simulink model "HeadwayControl_CleanedUpVFinal"  (R2018a)
settings: Solver=ode45  StartTime=0.0  StopTime=tsim  MaxStep=.1  RelTol=1e-3
values from neighbouring files (symbols this model uses):
  EndVel = (Time2-Time1)*Slope+StartVel    (= 31.525)    [ImpulseResponseStringStabilityV2.m]
  h = 2    [ImpulseResponseStringStabilityV2.m]
  InputNum = 3    [ImpulseResponseStringStabilityV2.m]
  InputTime = 1    [ImpulseResponseStringStabilityV2.m]
  lambda = 0.001    [ImpulseResponseStringStabilityV2.m]
  Slope = 0.5*g    (= 4.905)    [ImpulseResponseStringStabilityV2.m]
  StartVel = 7    [ImpulseResponseStringStabilityV2.m]
  tau = .5    (= 0.5)    [ImpulseResponseStringStabilityV2.m]
  Time1 = 2    [ImpulseResponseStringStabilityV2.m]
  Time2 = Time1 + DTime    (= 7)    [ImpulseResponseStringStabilityV2.m]
undefined symbols (not defined in the file or in its folder): heaviside
libraries: simulink x2
settings Model: Creator=domin  LastModifiedBy=domin

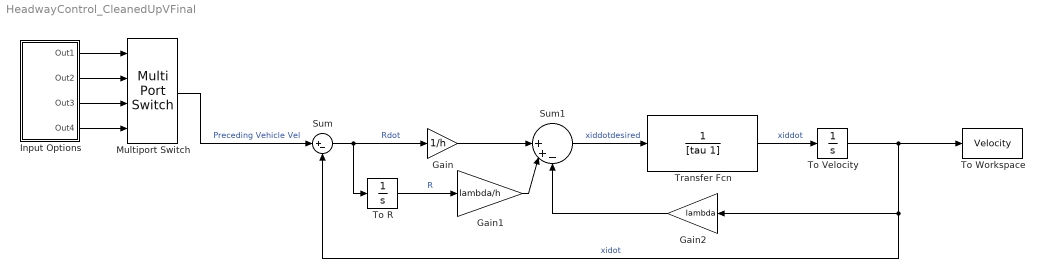
== system HeadwayControl_CleanedUpVFinal ==
  Gain : Gain  Gain=1/h
  Gain1 : Gain  Gain=lambda/h
  Gain2 : Gain  Gain=lambda
  Input Options : Subsystem
  Multiport Switch : MultiPortSwitch
  Sum : Sum  Inputs=|+-
  Sum1 : Sum  Inputs=||++-
  To R : Integrator  InitialCondition=h*StartVel
  To Velocity : Integrator  InitialCondition=StartVel
  To Workspace : ToWorkspace  VariableName=Velocity  SampleTime=-1
  Transfer Fcn : TransferFcn  Denominator=[tau 1]
  wires:
  Sum/1 -> To R/1, Gain/1  "Rdot"
  To R/1 -> Gain1/1  "R"
  Gain/1 -> Sum1/1
  Gain1/1 -> Sum1/2
  Sum1/1 -> Transfer Fcn/1  "xiddotdesired"
  Transfer Fcn/1 -> To Velocity/1  "xiddot"
  To Velocity/1 -> Sum/2, Gain2/1, To Workspace/1  "xidot"
  Gain2/1 -> Sum1/3
  Multiport Switch/1 -> Sum/1  "Preceding Vehicle Vel"
  Input Options/1(Out1) -> Multiport Switch/1
  Input Options/2(Out2) -> Multiport Switch/2
  Input Options/3(Out3) -> Multiport Switch/3
  Input Options/4(Out4) -> Multiport Switch/4

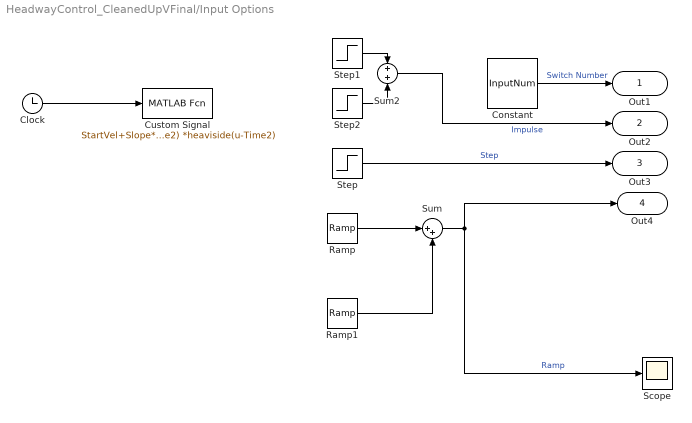
== system HeadwayControl_CleanedUpVFinal/Input Options ==
  Clock : Clock
  Constant : Constant  Value=InputNum
  Custom Signal : MATLABFcn  MATLABFcn=StartVel+Slope*(u-Time1) *heaviside(u-Time1)-Slope*(u-Time2) *heaviside(u-Time2)  OutputDimensions=1
  Ramp : simulink/Sources/Ramp  slope=Slope  start=Time1  InitialOutput=StartVel
  Ramp1 : simulink/Sources/Ramp  slope=-Slope  start=Time2  InitialOutput=0
  Scope : Scope
  Step : Step  Time=InputTime  Before=StartVel  After=EndVel  SampleTime=0
  Step1 : Step  Time=InputTime  Before=StartVel  After=StartVel+(1*10^10)  SampleTime=0
  Step2 : Step  Time=InputTime + (1*10^-10)  After=-(1*10^10)  SampleTime=0
  Sum : Sum  Inputs=|++
  Sum2 : Sum
  Out1 : Outport
  Out2 : Outport  Port=2
  Out3 : Outport  Port=3
  Out4 : Outport  Port=4
  wires:
  Clock/1 -> Custom Signal/1
  Sum2/1 -> Out2/1  "Impulse"
  Constant/1 -> Out1/1  "Switch Number"
  Step2/1 -> Sum2/2
  Step1/1 -> Sum2/1
  Step/1 -> Out3/1  "Step"
  Ramp/1 -> Sum/1
  Ramp1/1 -> Sum/2
  Sum/1 -> Out4/1, Scope/1  "Ramp"
